simulink model "arq2"  (R2013a)
settings: Solver=ode45  StartTime=0.0  StopTime=Tsim  RelTol=1e-3
values from neighbouring files (symbols this model uses):
  D = 4.1019    [load_variables.m]    (also in matlab.mat; matlab2.mat; matlab_workspace.mat)
  dist = 0    [CalibraQs.m]    (also in load_variables.m = 5; matlab.mat = 5; matlab2.mat = 5; matlab_workspace.mat = 5)
  I = 0.0044    [load_variables.m]    (also in matlab.mat; matlab2.mat; matlab_workspace.mat)
  P = 0.3105    [load_variables.m]    (also in matlab.mat; matlab2.mat; matlab_workspace.mat)
  ref = 10    [CalibraQs.m]    (also in load_variables.m; matlab.mat; matlab2.mat; matlab_workspace.mat)
  Tdist = 0    [CalibraQs.m]    (also in RenameVar.m = Tstep; matlab.mat = 1200; matlab2.mat = 1200; matlab_workspace.mat = 1400)
  Tdistdown = 0    [CalibraQs.m]    (also in RenameVar.m = Tstepdown; matlab.mat = 1800; matlab2.mat = 1800; matlab_workspace.mat = 1800)
  Tref = 800    [CalibraQs.m]    (also in load_variables.m; matlab.mat = 600; matlab2.mat = 600; matlab_workspace.mat = 700)
  Trefdown = Tref*2    (= 1600)    [CalibraQs.m]    (also in load_variables.m = 2420; matlab.mat = 2400; matlab2.mat = 2400; matlab_workspace.mat = 2500)
  Ts = 5    [load_variables.m]    (also in matlab.mat; matlab2.mat; matlab_workspace.mat)
  Tsim = Tref+Trefdown    (= 2400)    [CalibraQs.m]    (also in load_variables.m = 3220; matlab.mat = 800; matlab2.mat = 800; matlab_workspace.mat = 3200)
undefined symbols (not defined in the file): Td
libraries: cstblocks x5, opclib x3, simulink x2, commchan3 x1
settings Model: Creator=didaticontrol  LastModifiedBy=didaticontrol

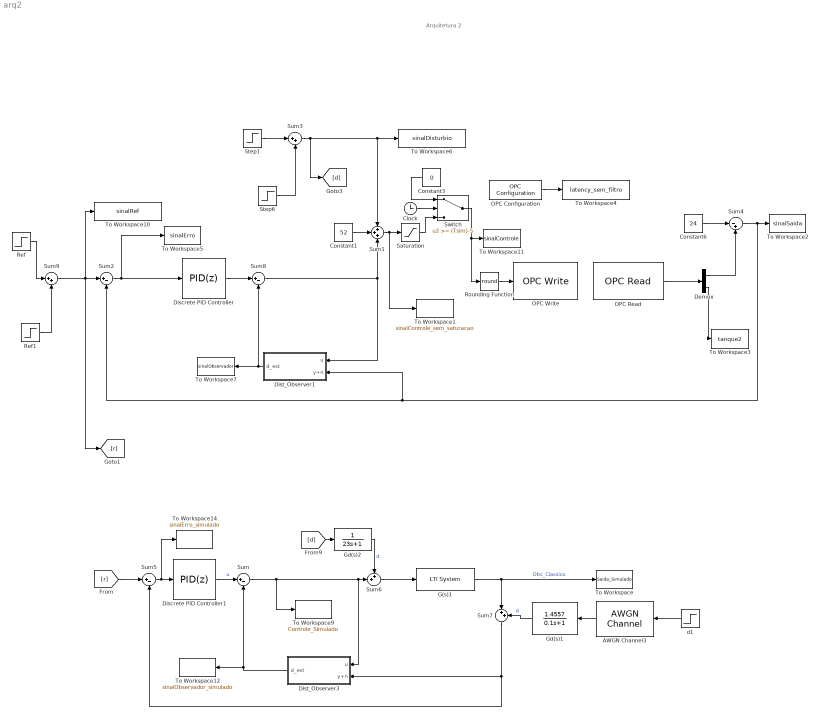
== system arq2 ==
  note: Arquitetura 2
  AWGN Channel3 : commchan3/AWGN Channel  InputProcessing=Columns as channels (frame based)  seed=67  noiseMode=Variance from mask  EbNodB=10  EsNodB=10  SNRdB=10  bitsPerSym=1  Ps=1  Tsym=1  variance=var_ruido
  Clock : Clock
  Constant1 : Constant  Value=52
  Constant3 : Constant  Value=0
  Constant6 : Constant  Value=24
  Demux : Demux  Outputs=2
  Discrete PID Controller : simulink/Continuous/PID Controller  Controller=PID  TimeDomain=Discrete-time  SampleTime=Ts  IntegratorMethod=Forward Euler  FilterMethod=Forward Euler  Form=Parallel  P=P  I=I  D=D  N=0  InitialConditionSource=internal  InitialConditionForIntegrator=0  InitialConditionForFilter=0  ExternalReset=none  LimitOutput=off  UpperSaturationLimit=inf  LowerSaturationLimit=-inf  LinearizeAsGain=off  AntiWindupMode=none  Kb=1  TrackingMode=off  Kt=1  PParamMin=[]  PParamMax=[]  IParamMin=[]  IParamMax=[]  DParamMin=[]  DParamMax=[]  NParamMin=[]  NParamMax=[]  KbParamMin=[]  KbParamMax=[]  KtParamMin=[]  KtParamMax=[]  POutMin=[]  POutMax=[]  IOutMin=[]  IOutMax=[]  DOutMin=[]  DOutMax=[]  NOutMin=[]  NOutMax=[]  KbOutMin=[]  KbOutMax=[]  KtOutMin=[]  KtOutMax=[]  IntegratorOutMin=[]  IntegratorOutMax=[]  FilterOutMin=[]  FilterOutMax=[]  SumOutMin=[]  SumOutMax=[]  SumI1OutMin=[]  SumI1OutMax=[]  SumI2OutMin=[]  SumI2OutMax=[]  SumI3OutMin=[]  SumI3OutMax=[]  SumDOutMin=[]  SumDOutMax=[]  SaturationOutMin=[]  SaturationOutMax=[]  IntegratorContinuousStateAttributes=''  IntegratorStateMustResolveToSignalObject=off  IntegratorRTWStateStorageClass=Auto  FilterContinuousStateAttributes=''  FilterStateMustResolveToSignalObject=off  FilterRTWStateStorageClass=Auto
  Discrete PID Controller1 : simulink/Continuous/PID Controller  Controller=PID  TimeDomain=Discrete-time  SampleTime=Ts  IntegratorMethod=Forward Euler  FilterMethod=Forward Euler  Form=Parallel  P=P  I=I  D=D  N=0  InitialConditionSource=internal  InitialConditionForIntegrator=0  InitialConditionForFilter=0  ExternalReset=none  LimitOutput=off  UpperSaturationLimit=inf  LowerSaturationLimit=-inf  LinearizeAsGain=off  AntiWindupMode=none  Kb=1  TrackingMode=off  Kt=1  PParamMin=[]  PParamMax=[]  IParamMin=[]  IParamMax=[]  DParamMin=[]  DParamMax=[]  NParamMin=[]  NParamMax=[]  KbParamMin=[]  KbParamMax=[]  KtParamMin=[]  KtParamMax=[]  POutMin=[]  POutMax=[]  IOutMin=[]  IOutMax=[]  DOutMin=[]  DOutMax=[]  NOutMin=[]  NOutMax=[]  KbOutMin=[]  KbOutMax=[]  KtOutMin=[]  KtOutMax=[]  IntegratorOutMin=[]  IntegratorOutMax=[]  FilterOutMin=[]  FilterOutMax=[]  SumOutMin=[]  SumOutMax=[]  SumI1OutMin=[]  SumI1OutMax=[]  SumI2OutMin=[]  SumI2OutMax=[]  SumI3OutMin=[]  SumI3OutMax=[]  SumDOutMin=[]  SumDOutMax=[]  SaturationOutMin=[]  SaturationOutMax=[]  IntegratorContinuousStateAttributes=''  IntegratorStateMustResolveToSignalObject=off  IntegratorRTWStateStorageClass=Auto  FilterContinuousStateAttributes=''  FilterStateMustResolveToSignalObject=off  FilterRTWStateStorageClass=Auto
  Dist_Observer1 : Subsystem  mask{Td=Td}
      mask prompts: Td "Filter time cte (Td)"
  Dist_Observer3 : Subsystem  mask{Td=Td}
      mask prompts: Td "Filter time cte (Td)"
  G(s)1 : cstblocks/LTI System  sys=Gs  IC=[]
  Gd(s)1 : TransferFcn  Numerator=1.4557  Denominator=[0.1 1]
  Gd(s)2 : TransferFcn  Numerator=1  Denominator=[23 1]
  OPC Configuration : opclib/OPC Configuration  opcServers=143.106.123.105/BR.OPC.Server_AR/10  errMissingItems=Error  errReadWrite=Warn  errShutdown=Error  errRTViolation=Warn  rtEnable=on  speedup=1  showLatency=on  beingUsed=on
  OPC Read : opclib/OPC Read  serverHost=143.106.123.105  serverID=BR.OPC.Server_AR  itemIDs=PTQ4_corrigido, PTQ2_corrigido  readMode=Synchronous (cache)  dataType=double  updateRate=5  showQual=off  showTS=off  tsMode=Seconds since start
  OPC Write : opclib/OPC Write  serverHost=143.106.123.105  serverID=BR.OPC.Server_AR  itemIDs=Bomba2  writeMode=Synchronous  updateRate=-1
  Ref : Step  Time=Tref  After=ref  SampleTime=0
  Ref1 : Step  Time=Trefdown  After=-ref  SampleTime=0
  Rounding Function : Rounding  Operator=round
  Saturation : Saturate  UpperLimit=80  LowerLimit=0
  Step1 : Step  Time=Tdist  After=dist  SampleTime=0
  Step6 : Step  Time=Tdistdown  After=-dist  SampleTime=0
  Sum{,2,5,8} (4 alike) : Sum  Inputs=|+-
  Sum1 : Sum  Inputs=+++
  Sum3 : Sum  Inputs=|++
  Sum4 : Sum  Inputs=|-+
  Sum6 : Sum  Inputs=++|
  Sum7 : Sum  Inputs=|++
  Sum9 : Sum  Inputs=|++
  Switch : Switch  Threshold=(Tsim)-5
  To Workspace : ToWorkspace  VariableName=Saida_Simulado  SampleTime=-1  SaveFormat=Timeseries
  To Workspace1 : ToWorkspace  VariableName=sinalControle_sem_saturacao  SampleTime=Ts  SaveFormat=Timeseries
  To Workspace10 : ToWorkspace  VariableName=sinalRef  SampleTime=Ts  SaveFormat=Timeseries
  To Workspace11 : ToWorkspace  VariableName=sinalControle  SampleTime=Ts  SaveFormat=Timeseries
  To Workspace12 : ToWorkspace  VariableName=sinalObservador_simulado  SampleTime=Ts  SaveFormat=Timeseries
  To Workspace14 : ToWorkspace  VariableName=sinalErro_simulado  SampleTime=Ts  SaveFormat=Timeseries
  To Workspace2 : ToWorkspace  VariableName=sinalSaida  SampleTime=Ts  SaveFormat=Timeseries
  To Workspace3 : ToWorkspace  VariableName=tanque2  SampleTime=Ts  SaveFormat=Timeseries
  To Workspace4 : ToWorkspace  VariableName=latency_sem_filtro  SampleTime=Ts  SaveFormat=Timeseries
  To Workspace5 : ToWorkspace  VariableName=sinalErro  SampleTime=Ts  SaveFormat=Timeseries
  To Workspace6 : ToWorkspace  VariableName=sinalDisturbio  SampleTime=Ts  SaveFormat=Timeseries
  To Workspace7 : ToWorkspace  VariableName=sinalObservador  SampleTime=Ts  SaveFormat=Timeseries
  To Workspace9 : ToWorkspace  VariableName=Controle_Simulado  SampleTime=-1  SaveFormat=Timeseries
  d1 : Step  Time=0  After=0  SampleTime=Ts
  wires:
  Constant6/1 -> Sum4/1
  OPC Read/1 -> Demux/1
  Demux/1 -> Sum4/2
  Demux/2 -> To Workspace3/1
  OPC Configuration/1 -> To Workspace4/1
  Step6/1 -> Sum3/2
  Step1/1 -> Sum3/1
  Constant1/1 -> Sum1/2
  Rounding Function/1 -> OPC Write/1
  Sum6/1 -> G(s)1/1
  Sum5/1 -> To Workspace14/1, Discrete PID Controller1/1
  Discrete PID Controller1/1 -> Sum/1  "u"
  Sum/1 -> To Workspace9/1, Dist_Observer3/1(u), Sum6/2
  Gd(s)2/1 -> Sum6/1  "d"
  Discrete PID Controller/1 -> Sum8/1
  Sum8/1 -> Sum1/3, Dist_Observer1/1(u)
  Sum4/1 -> Dist_Observer1/2(y+n), Sum2/2, To Workspace2/1
  Dist_Observer1/1(d_est) -> To Workspace7/1, Sum8/2
  Switch/1 -> To Workspace11/1, Rounding Function/1
  Clock/1 -> Switch/2
  Constant3/1 -> Switch/1
  Ref/1 -> Sum9/1
  Ref1/1 -> Sum9/2
  Saturation/1 -> Switch/3
  Dist_Observer3/1(d_est) -> To Workspace12/1, Sum/2
  Sum2/1 -> Discrete PID Controller/1, To Workspace5/1
  Sum1/1 -> To Workspace1/1, Saturation/1
  Sum9/1 -> [r], Sum2/1, To Workspace10/1
  [r] -> Sum5/1
  Sum7/1 -> Sum5/2, Dist_Observer3/2(y+n)
  d1/1 -> AWGN Channel3/1
  AWGN Channel3/1 -> Gd(s)1/1
  Gd(s)1/1 -> Sum7/2  "d"
  G(s)1/1 -> To Workspace/1, Sum7/1  "Obs_Classico"
  [d] -> Gd(s)2/1
  Sum3/1 -> Sum1/1, To Workspace6/1, [d]

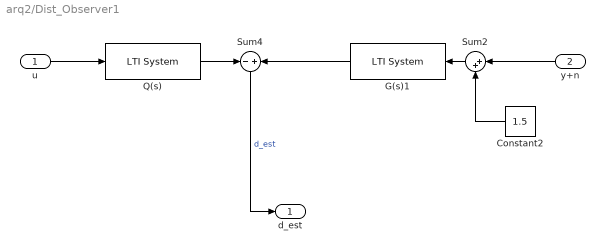
== system arq2/Dist_Observer1 ==
  u : Inport
  y+n : Inport  Port=2
  Constant2 : Constant  Value=1.5
  G(s)1 : cstblocks/LTI System  sys=G_inv_Q  IC=[]
  Q(s) : cstblocks/LTI System  sys=Qs  IC=[]
  Sum2 : Sum  Inputs=|++
  Sum4 : Sum  Inputs=-|+
  d_est : Outport
  wires:
  Q(s)/1 -> Sum4/1
  Sum4/1 -> d_est/1  "d_est"
  Sum2/1 -> G(s)1/1
  u/1 -> Q(s)/1
  Constant2/1 -> Sum2/2
  y+n/1 -> Sum2/1
  G(s)1/1 -> Sum4/2

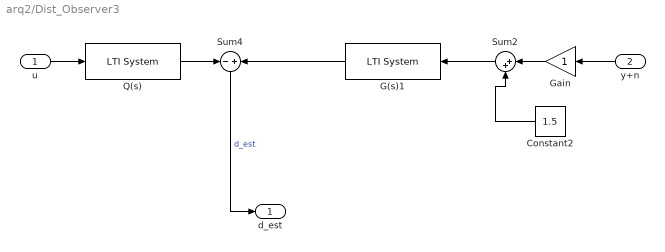
== system arq2/Dist_Observer3 ==
  u : Inport
  y+n : Inport  Port=2
  Constant2 : Constant  Value=1.5
  G(s)1 : cstblocks/LTI System  sys=G_inv_Q  IC=[]
  Gain : Gain
  Q(s) : cstblocks/LTI System  sys=Qs  IC=[]
  Sum2 : Sum  Inputs=|++
  Sum4 : Sum  Inputs=-|+
  d_est : Outport
  wires:
  Q(s)/1 -> Sum4/1
  Sum4/1 -> d_est/1  "d_est"
  u/1 -> Q(s)/1
  G(s)1/1 -> Sum4/2
  Sum2/1 -> G(s)1/1
  Constant2/1 -> Sum2/2
  Gain/1 -> Sum2/1
  y+n/1 -> Gain/1
